simulink model "pv_model_2sx1p_final"  (R2017b)
settings: Solver=ode23tb  StartTime=0.0  StopTime=1.5  MaxStep=1e-4  RelTol=1e-4  AbsTol=1e-5  EnableMultiTasking=on
InitFcn:
  | Nss = str2num(get_param([gcs,'/Nss_'],'Value'));
  | Npp = str2num(get_param([gcs,'/Npp_'],'Value'));
  | G = str2num(get_param([gcs,'/G_'],'Value'));
  | T = str2num(get_param([gcs,'/T_'],'Value'));
  | Rs = Rsn;
  | Rp = (Gn/G)*Rpn;
values from neighbouring files (symbols this model uses):
  a = an    (= 1.3)    [PVCurvePlot_2sx1p.m]
  Gn = 1000    [PVCurvePlot_2sx1p.m]
undefined symbols (not defined in the file or in its folder): a_n, ILn, Iscn, k, Ki, Kv, Ns, q, Rpn, Rsn, T_n, Tn, Vocn
libraries: powerlib x31, simulink x2
settings Model: Creator=marcelo  LastModifiedBy=Ceyhun
settings SolverCC: SolverResetMethod=Robust
settings DataIOCC: LimitDataPoints=on  SaveFormat=Array  SignalLoggingSaveFormat=ModelDataLogs
settings OptimizationCC: ExpressionDepthLimit=2147483647  InitFltsAndDblsToZero=on  LifeSpan=inf
settings DebuggingCC: SaveWithParameterizedLinksMsg=none  UnderspecifiedInitializationDetection=Classic  MergeDetectMultiDrivingBlocksExec=none  SignalResolutionControl=TryResolveAllWithWarning  SolverPrmCheckMsg=warning  FcnCallInpInsideContextMsg=warning  StateNameClashWarn=warning  SFUnexpectedBacktrackingDiag=warning  SFNoUnconditionalDefaultTransitionDiag=warning  SFExecutionAtInitializationDiag=none
settings HardwareCC: ProdBitPerPointer=32  ProdBitPerSizeT=32  ProdBitPerPtrDiffT=32  ProdLargestAtomicFloat=None  ProdIntDivRoundTo=Undefined  ProdEndianess=Unspecified  ProdWordSize=32  ProdHWDeviceType=32-bit Generic
settings ModelReferenceCC: PropagateSignalLabelsOutOfModel=off
settings CodeAppCC: StateflowObjectComments=on
settings GRTTargetCC: TargetFcnLib=ansi_tfl_tmw.mat  TargetLangStandard=C89/C90 (ANSI)  GeneratePreprocessorConditionals=Disable all  CombineOutputUpdateFcns=off  GRTInterface=on
settings ConfigComp: CovMetricSettings=dw  CovHtmlReporting=on  CovSaveCumulativeToWorkspaceVar=on  CovSaveSingleToWorkspaceVar=on  CovExternalEMLEnable=off
settings SimscapeCC: SimscapeNormalizeSystem=off

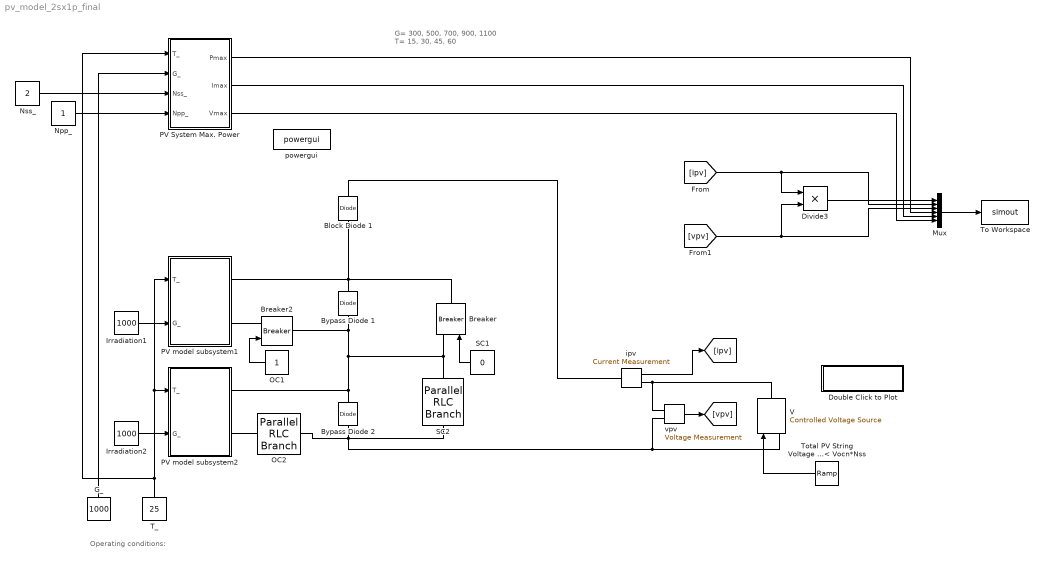
== system pv_model_2sx1p_final ==
  note: G= 300, 500, 700, 900, 1100
      | T= 15, 30, 45, 60
  note: Operating conditions:
  Block Diode 1 : powerlib/Power Electronics/Diode  Ron=0.001  Lon=0  Vf=0.8  IC=0  UseSnubber=off  Rs=500  Cs=250e-9  Measurements=off
  Breaker : powerlib/Elements/Breaker  InitialState=0  SwitchingTimes="[1/60  5/60]"  External=on  BreakerResistance=0.01  SnubberResistance=1e9  SnubberCapacitance=inf  Measurements=None  MoreParameters=on  NoBreakLoop=off
      settings: SourceProductName=Simscape Power Systems
  Breaker2 : powerlib/Elements/Breaker  InitialState=0  SwitchingTimes="[1/60  5/60]"  External=on  BreakerResistance=0.01  SnubberResistance=1e9  SnubberCapacitance=inf  Measurements=None  MoreParameters=on  NoBreakLoop=off
      settings: SourceProductName=Simscape Power Systems
  Bypass Diode 1 : powerlib/Power Electronics/Diode  Ron=0.001  Lon=0  Vf=0.8  IC=0  UseSnubber=off  Rs=500  Cs=250e-9  Measurements=off
  Bypass Diode 2 : powerlib/Power Electronics/Diode  Ron=0.001  Lon=0  Vf=0.8  IC=0  UseSnubber=off  Rs=500  Cs=250e-9  Measurements=off
  Divide3 : Product  Inputs=**
  Double Click to Plot : Subsystem
      settings: OpenFcn=PVCurvePlot_2sx1p
      mask Display: disp('Plot PV Curve');
  G_ : Constant  Value=1000
  Irradiation1 : Constant  Value=1000
  Irradiation2 : Constant  Value=1000
  Mux : Mux  Inputs=6
  Npp_ : Constant
  Nss_ : Constant  Value=2
  OC1 : Constant
  OC2 : powerlib/Elements/Parallel RLC Branch  LConnTagsString=a  RConnTagsString=__new0  BranchType=R  Resistance=0.01  Inductance=1e-3  SetiL0=off  InitialCurrent=0  Capacitance=1e-6  Setx0=off  InitialVoltage=0  Measurements=None
  PV System Max. Power : Subsystem
  PV model subsystem1 : Subsystem
  PV model subsystem2 : Subsystem
  SC1 : Constant  Value=0
  SC2 : powerlib/Elements/Parallel RLC Branch  LConnTagsString=a  RConnTagsString=__new0  BranchType=R  Resistance=1e9  Inductance=1e-3  SetiL0=off  InitialCurrent=0  Capacitance=1e-6  Setx0=off  InitialVoltage=0  Measurements=None
  T_ : Constant  Value=25
  To Workspace : ToWorkspace  VariableName=simout  SampleTime=-1
  Total PV String Voltage 0 < V < Vocn*Nss : simulink/Sources/Ramp  slope=Vocn*2  start=0  X0=0
  V : powerlib/Electrical Sources/Controlled Voltage Source  Initialize=on  Source_Type=DC  Amplitude=0  Phase=0  Frequency=0  Measurements=None
  ipv : powerlib/Measurements/Current Measurement  PhasorSimulation=off  OutputType=Complex  PSBequivalent=0
  powergui : powerlib/powergui  SimulationMode=Continuous  SampleTime=1e-4  frequency=60  Iterations=50  frequencyindice=0  Pbase=100e6  ErrMax=1e-4  UnitsV=kV  UnitsW=MW  buscounter=0  FunctionMessages=off  echomessages=off  EnableUseOfTLC=off  CurrentSourceSwitches=off  DisableSnubberDevices=off  DisableRonSwitches=off  DisableVfSwitches=off  DisplayEquations=off  SolverType=Tustin/Backward Euler (TBE)  Interpol=off  ExternalGateDelay=off  methode=off  Ts=100  x0status=blocks  SPID=on  SwTol=0  HookPort=off  RestoreLinks=warning  ResistiveCurrentMeasurement=off  Frange=[0:2:500]  Ylog=off  Xlog=on  ShowGrid=off  save=off  variable=ZData  structure=0  ZoomFFT=on  StartTime=0.0  cycles=1  DisplayStyle=1  fundamental=60  FreqAxis=off  MaxFrequency=1000  frequencyindicesteady=1  RmsSteady=1  display=off
  vpv : powerlib/Measurements/Voltage Measurement  PhasorSimulation=off  OutputType=Complex  PSBequivalent=0
  wires:
  Total PV String Voltage 0 < V < Vocn*Nss/1 -> V/1
  ipv/1 -> [ipv]
  vpv/1 -> [vpv]
  T_/1 -> PV model subsystem2/1(T_), PV model subsystem1/1(T_), PV System Max. Power/1(T_)
  Irradiation1/1 -> PV model subsystem1/2(G_)
  Irradiation2/1 -> PV model subsystem2/2(G_)
  [ipv] -> Mux/2, Divide3/1
  [vpv] -> Divide3/2, Mux/3
  Divide3/1 -> Mux/1
  Mux/1 -> To Workspace/1
  Nss_/1 -> PV System Max. Power/3(Nss_)
  Npp_/1 -> PV System Max. Power/4(Npp_)
  G_/1 -> PV System Max. Power/2(G_)
  PV System Max. Power/1(Pmax) -> Mux/4
  PV System Max. Power/2(Imax) -> Mux/5
  PV System Max. Power/3(Vmax) -> Mux/6
  SC1/1 -> Breaker/1
  OC1/1 -> Breaker2/1
  connections:
  ipv/RConn1 -- V/RConn1 -- vpv/LConn1
  Bypass Diode 1/RConn1 -- Breaker/RConn1 -- PV model subsystem1/RConn1 -- Block Diode 1/LConn1
  V/LConn1 -- SC2/LConn1 -- OC2/RConn1 -- Bypass Diode 2/LConn1 -- vpv/LConn2
  Bypass Diode 2/RConn1 -- PV model subsystem2/RConn1 -- Breaker2/RConn1 -- Bypass Diode 1/LConn1 -- Breaker/LConn1 -- SC2/RConn1
  Breaker2/LConn1 -- PV model subsystem1/RConn2
  PV model subsystem2/RConn2 -- OC2/LConn1
  Block Diode 1/RConn1 -- ipv/LConn1

== system pv_model_2sx1p_final/Double Click to Plot ==

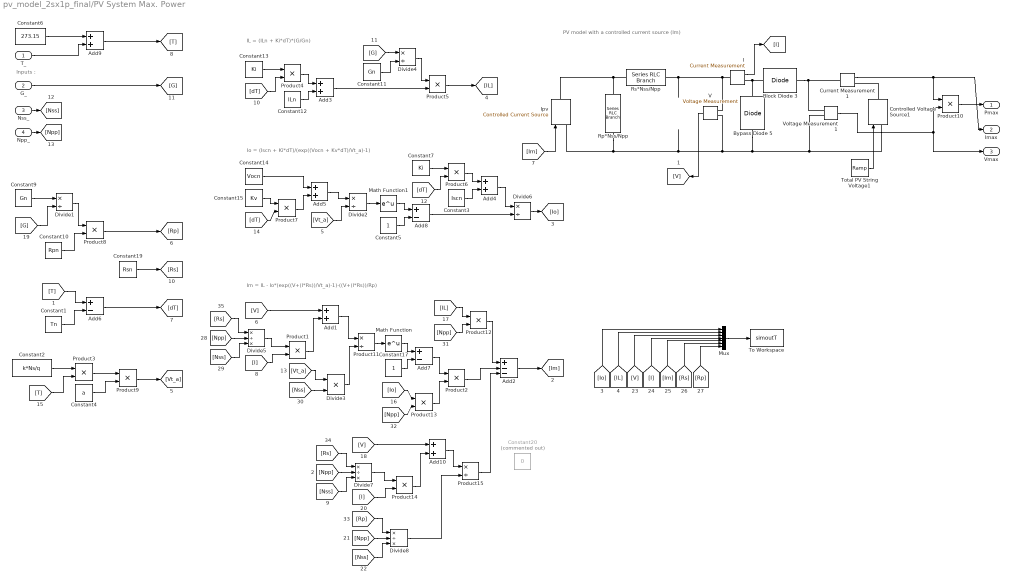
== system pv_model_2sx1p_final/PV System Max. Power ==
  note: Im = IL - Io*(exp((V+(I*Rs))/Vt_a)-1)-((V+(I*Rs))/Rp)
  note: Inputs :
  note: Io = (Iscn + Ki*dT)/(exp((Vocn + Kv*dT)/Vt_a)-1)
  note: PV model with a controlled current source (Im)
  note: IL = (ILn + Ki*dT)*(G/Gn)
  T_ : Inport
  G_ : Inport  Port=2
  Nss_ : Inport  Port=3
  Npp_ : Inport  Port=4
  Add{1,3..5,9..10} (6 alike) : Sum
  Add2 : Sum  Inputs=+--
  Add6 : Sum  Inputs=+-
  Add7 : Sum  Inputs=+-
  Add8 : Sum  Inputs=+-
  Block Diode 3 : powerlib/Power Electronics/Diode  Ron=0.001  Lon=0  Vf=0.8  IC=0  UseSnubber=off  Rs=500  Cs=250e-9  Measurements=off
  Bypass Diode 5 : powerlib/Power Electronics/Diode  Ron=0.001  Lon=0  Vf=0.8  IC=0  UseSnubber=off  Rs=500  Cs=250e-9  Measurements=off
  Constant1 : Constant  Value=Tn
  Constant10 : Constant  Value=Rpn
  Constant11 : Constant  Value=Gn
  Constant12 : Constant  Value=ILn
  Constant13 : Constant  Value=Ki
  Constant14 : Constant  Value=Vocn
  Constant15 : Constant  Value=Kv
  Constant17 : Constant
  Constant19 : Constant  Value=Rsn
  Constant2 : Constant  Value=k*Ns/q
  Constant20 : Constant  Commented=on  Value=0
  Constant3 : Constant  Value=Iscn
  Constant4 : Constant  Value=a
  Constant5 : Constant
  Constant6 : Constant  Value=273.15
  Constant7 : Constant  Value=Ki
  Constant9 : Constant  Value=Gn
  Controlled Voltage Source1 : powerlib/Electrical Sources/Controlled Voltage Source  Initialize=on  Source_Type=DC  Amplitude=0  Phase=0  Frequency=0  Measurements=None
  Current Measurement1 : powerlib/Measurements/Current Measurement  PhasorSimulation=off  OutputType=Complex  PSBequivalent=0
  Divide{1..2,4,6} (4 alike) : Product  Inputs=*/
  Divide3 : Product
  Divide5 : Product  Inputs=*/*
  Divide7 : Product  Inputs=*/*
  Divide8 : Product  Inputs=*/*
  I : powerlib/Measurements/Current Measurement  PhasorSimulation=off  OutputType=Complex  PSBequivalent=0
  Ipv : powerlib/Electrical Sources/Controlled Current Source  Initialize=on  Source_Type=DC  Amplitude=0  Phase=0  Frequency=0  Measurements=None
  Math Function : Math  SaturateOnIntegerOverflow=on
  Math Function1 : Math  SaturateOnIntegerOverflow=on
  Mux : Mux  Inputs=7
  Product{1..9,12..14} (12 alike) : Product  RndMeth=Zero
  Product10 : Product
  Product11 : Product  Inputs=*/  RndMeth=Zero
  Product15 : Product  Inputs=*/  RndMeth=Zero
  Rp*Nss/Npp : powerlib/Elements/Series RLC Branch  LConnTagsString=__new0  RConnTagsString=__new0  BranchType=R  Resistance=Rp*Nss/Npp  Inductance=1e-3  SetiL0=off  InitialCurrent=0  Capacitance=1e-6  Setx0=off  InitialVoltage=0  Measurements=None
  Rs*Nss/Npp : powerlib/Elements/Series RLC Branch  LConnTagsString=__new0  RConnTagsString=__new0  BranchType=R  Resistance=Rs*Nss/Npp  Inductance=1e-3  SetiL0=off  InitialCurrent=0  Capacitance=1e-6  Setx0=off  InitialVoltage=0  Measurements=None
  To Workspace : ToWorkspace  VariableName=simoutT  SampleTime=-1
  Total PV String Voltage1 : simulink/Sources/Ramp  slope=Vocn*Nss  start=0  X0=0
  "V " : powerlib/Measurements/Voltage Measurement  PhasorSimulation=off  OutputType=Complex  PSBequivalent=0
  Voltage Measurement1 : powerlib/Measurements/Voltage Measurement  PhasorSimulation=off  OutputType=Complex  PSBequivalent=0
  Pmax : Outport
  Imax : Outport  Port=2
  Vmax : Outport  Port=3
  wires:
  I/1 -> [I]
  "V "/1 -> [V]
  [Im] -> Ipv/1
  G_/1 -> [G]
  [I] -> Product1/2
  [V] -> Add1/1
  Add2/1 -> [Im]
  [G] -> Divide4/1
  Constant11/1 -> Divide4/2
  Constant13/1 -> Product4/1
  [dT] -> Product6/2
  Constant7/1 -> Product6/1
  [dT] -> Product7/2
  Constant14/1 -> Add5/1
  Divide2/1 -> Math Function1/1
  Add5/1 -> Divide2/1
  Constant17/1 -> Add7/2
  Add7/1 -> Product2/1
  Constant5/1 -> Add8/2
  Math Function1/1 -> Add8/1
  Divide6/1 -> [Io]
  Product5/1 -> [IL]
  Product1/1 -> Add1/2
  Math Function/1 -> Add7/1
  Product4/1 -> Add3/1
  Add3/1 -> Product5/2
  Divide4/1 -> Product5/1
  Product7/1 -> Add5/2
  Constant15/1 -> Product7/1
  Add8/1 -> Divide6/2
  Constant3/1 -> Add4/2
  Product6/1 -> Add4/1
  Constant12/1 -> Add3/2
  Product2/1 -> Add2/2
  [dT] -> Product4/2
  Add4/1 -> Divide6/1
  Mux/1 -> To Workspace/1
  [Io] -> Mux/1
  [IL] -> Mux/2
  Add6/1 -> [dT]
  [T] -> Add6/1
  Constant1/1 -> Add6/2
  Constant2/1 -> Product3/1
  [Rs] -> Mux/6
  Divide1/1 -> Product8/1
  Product8/1 -> [Rp]
  Constant10/1 -> Product8/2
  Add9/1 -> [T]
  [Im] -> Mux/5
  [I] -> Mux/4
  [V] -> Mux/3
  [Vt_a] -> Divide2/2
  Constant4/1 -> Product9/2
  Product3/1 -> Product9/1
  Product9/1 -> [Vt_a]
  [T] -> Product3/2
  Constant9/1 -> Divide1/1
  [G] -> Divide1/2
  T_/1 -> Add9/2
  Constant6/1 -> Add9/1
  [Rp] -> Mux/7
  Constant19/1 -> [Rs]
  [Rs] -> Divide5/1
  Divide5/1 -> Product1/1
  [Npp] -> Divide5/2
  [Nss] -> Divide5/3
  [Vt_a] -> Divide3/1
  [IL] -> Product12/1
  [Npp] -> Product12/2
  Product12/1 -> Add2/1
  [Io] -> Product13/1
  [Npp] -> Product13/2
  Product13/1 -> Product2/2
  Npp_/1 -> [Npp]
  Nss_/1 -> [Nss]
  Voltage Measurement1/1 -> Vmax/1, Product10/2
  Product10/1 -> Pmax/1
  Current Measurement1/1 -> Imax/1, Product10/1
  Total PV String Voltage1/1 -> Controlled Voltage Source1/1
  Product11/1 -> Math Function/1
  Divide3/1 -> Product11/2
  Add1/1 -> Product11/1
  [Nss] -> Divide3/2
  Divide8/1 -> Product15/2
  [Nss] -> Divide7/3
  [Npp] -> Divide7/2
  Product14/1 -> Add10/2
  [I] -> Product14/2
  [Rs] -> Divide7/1
  [V] -> Add10/1
  [Nss] -> Divide8/3
  Divide7/1 -> Product14/1
  Add10/1 -> Product15/1
  [Rp] -> Divide8/1
  [Npp] -> Divide8/2
  Product15/1 -> Add2/3
  connections:
  I/LConn1 -- Rs*Nss/Npp/RConn1 -- "V "/LConn1
  Ipv/RConn1 -- Rs*Nss/Npp/LConn1 -- Rp*Nss/Npp/LConn1
  Controlled Voltage Source1/LConn1 -- Voltage Measurement1/LConn2 -- Bypass Diode 5/LConn1 -- Rp*Nss/Npp/RConn1 -- Ipv/LConn1 -- "V "/LConn2
  Controlled Voltage Source1/RConn1 -- Current Measurement1/RConn1
  Voltage Measurement1/LConn1 -- Current Measurement1/LConn1 -- Block Diode 3/RConn1
  Block Diode 3/LConn1 -- Bypass Diode 5/RConn1 -- I/RConn1

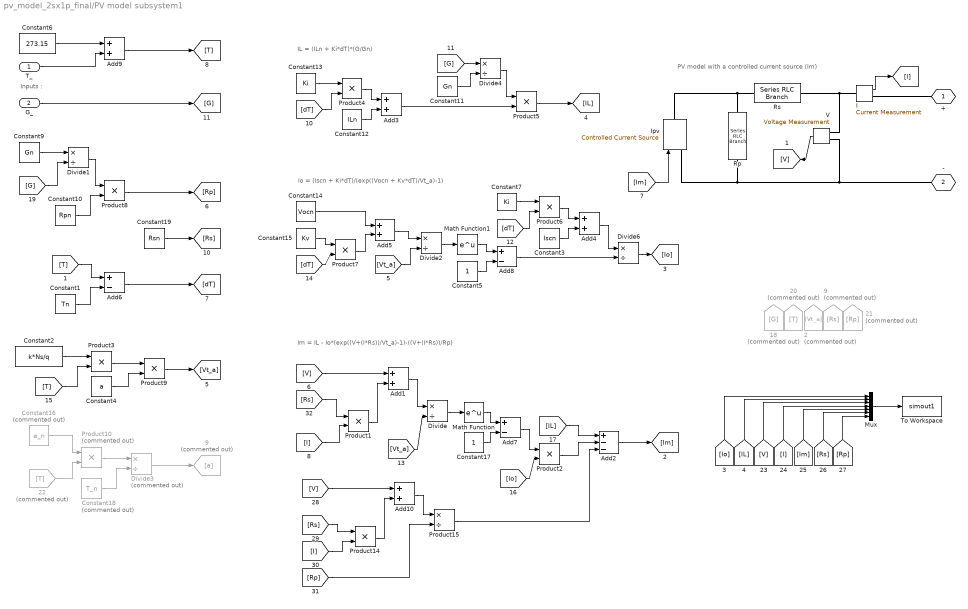
== system pv_model_2sx1p_final/PV model subsystem1 ==
  note: Im = IL - Io*(exp((V+(I*Rs))/Vt_a)-1)-((V+(I*Rs))/Rp)
  note: Inputs :
  note: Io = (Iscn + Ki*dT)/(exp((Vocn + Kv*dT)/Vt_a)-1)
  note: PV model with a controlled current source (Im)
  note: IL = (ILn + Ki*dT)*(G/Gn)
  T_ : Inport
  G_ : Inport  Port=2
  "       9" : Goto  Commented=on  GotoTag=a
  "   18" : From  Commented=on  GotoTag=G
      settings: CloseFcn=tagdialog Close
  "   2" : From  Commented=on  GotoTag=Vt_a
      settings: CloseFcn=tagdialog Close
  "   20" : From  Commented=on  GotoTag=T
      settings: CloseFcn=tagdialog Close
  "   21" : From  Commented=on  GotoTag=Rp
      settings: CloseFcn=tagdialog Close
  "   22" : From  Commented=on  GotoTag=T
      settings: CloseFcn=tagdialog Close
  "   9" : From  Commented=on  GotoTag=Rs
      settings: CloseFcn=tagdialog Close
  Add{1,3..5,9..10} (6 alike) : Sum
  Add2 : Sum  Inputs=+--
  Add6 : Sum  Inputs=+-
  Add7 : Sum  Inputs=+-
  Add8 : Sum  Inputs=+-
  Constant1 : Constant  Value=Tn
  Constant10 : Constant  Value=Rpn
  Constant11 : Constant  Value=Gn
  Constant12 : Constant  Value=ILn
  Constant13 : Constant  Value=Ki
  Constant14 : Constant  Value=Vocn
  Constant15 : Constant  Value=Kv
  Constant16 : Constant  Commented=on  Value=a_n
  Constant17 : Constant
  Constant18 : Constant  Commented=on  Value=T_n
  Constant19 : Constant  Value=Rsn
  Constant2 : Constant  Value=k*Ns/q
  Constant3 : Constant  Value=Iscn
  Constant4 : Constant  Value=a
  Constant5 : Constant
  Constant6 : Constant  Value=273.15
  Constant7 : Constant  Value=Ki
  Constant9 : Constant  Value=Gn
  Divide{,1..2,4,6} (5 alike) : Product  Inputs=*/
  Divide3 : Product  Commented=on  Inputs=*/
  I : powerlib/Measurements/Current Measurement  PhasorSimulation=off  OutputType=Complex  PSBequivalent=0
  Ipv : powerlib/Electrical Sources/Controlled Current Source  Initialize=on  Source_Type=DC  Amplitude=0  Phase=0  Frequency=0  Measurements=None
  Math Function : Math  SaturateOnIntegerOverflow=on
  Math Function1 : Math  SaturateOnIntegerOverflow=on
  Mux : Mux  Inputs=7
  Product{1..9,14} (10 alike) : Product  RndMeth=Zero
  Product10 : Product  Commented=on  RndMeth=Zero
  Product15 : Product  Inputs=*/  RndMeth=Zero
  Rp : powerlib/Elements/Series RLC Branch  LConnTagsString=__new0  RConnTagsString=__new0  BranchType=R  Resistance=Rp  Inductance=1e-3  SetiL0=off  InitialCurrent=0  Capacitance=1e-6  Setx0=off  InitialVoltage=0  Measurements=None
  Rs : powerlib/Elements/Series RLC Branch  LConnTagsString=__new0  RConnTagsString=__new0  BranchType=R  Resistance=Rs  Inductance=1e-3  SetiL0=off  InitialCurrent=0  Capacitance=1e-6  Setx0=off  InitialVoltage=0  Measurements=None
  To Workspace : ToWorkspace  VariableName=simout1  SampleTime=-1
  "V " : powerlib/Measurements/Voltage Measurement  PhasorSimulation=off  OutputType=Complex  PSBequivalent=0
  + : PMIOPort  Port=1  Side=Right
  - : PMIOPort  Port=2  Side=Right
  wires:
  I/1 -> [I]
  "V "/1 -> [V]
  [Im] -> Ipv/1
  G_/1 -> [G]
  [I] -> Product1/2
  [V] -> Add1/1
  Divide/1 -> Math Function/1
  Add2/1 -> [Im]
  Add1/1 -> Divide/1
  [G] -> Divide4/1
  Constant11/1 -> Divide4/2
  Constant13/1 -> Product4/1
  [dT] -> Product6/2
  Constant7/1 -> Product6/1
  [dT] -> Product7/2
  Constant14/1 -> Add5/1
  Divide2/1 -> Math Function1/1
  Add5/1 -> Divide2/1
  Constant17/1 -> Add7/2
  Add7/1 -> Product2/1
  Constant5/1 -> Add8/2
  Math Function1/1 -> Add8/1
  Divide6/1 -> [Io]
  Product5/1 -> [IL]
  Product1/1 -> Add1/2
  Math Function/1 -> Add7/1
  Product4/1 -> Add3/1
  Add3/1 -> Product5/2
  Divide4/1 -> Product5/1
  Product7/1 -> Add5/2
  Constant15/1 -> Product7/1
  Add8/1 -> Divide6/2
  Constant3/1 -> Add4/2
  Product6/1 -> Add4/1
  Constant12/1 -> Add3/2
  Product2/1 -> Add2/2
  [Io] -> Product2/2
  [IL] -> Add2/1
  [Rs] -> Product1/1
  [dT] -> Product4/2
  Add4/1 -> Divide6/1
  Mux/1 -> To Workspace/1
  [Io] -> Mux/1
  [IL] -> Mux/2
  Add6/1 -> [dT]
  [T] -> Add6/1
  Constant1/1 -> Add6/2
  Constant2/1 -> Product3/1
  [Rs] -> Mux/6
  Divide1/1 -> Product8/1
  Product8/1 -> [Rp]
  Constant10/1 -> Product8/2
  Add9/1 -> [T]
  [Im] -> Mux/5
  [I] -> Mux/4
  [V] -> Mux/3
  [Vt_a] -> Divide2/2
  [Vt_a] -> Divide/2
  Constant4/1 -> Product9/2
  Product3/1 -> Product9/1
  Product9/1 -> [Vt_a]
  [T] -> Product3/2
  Constant9/1 -> Divide1/1
  [G] -> Divide1/2
  T_/1 -> Add9/2
  Constant6/1 -> Add9/1
  Constant16/1 -> Product10/1
  "   22"/1 -> Product10/2
  Product10/1 -> Divide3/1
  Constant18/1 -> Divide3/2
  Divide3/1 -> "       9"/1
  [Rp] -> Mux/7
  Constant19/1 -> [Rs]
  [Rp] -> Product15/2
  Product14/1 -> Add10/2
  [I] -> Product14/2
  [V] -> Add10/1
  [Rs] -> Product14/1
  Product15/1 -> Add2/3
  Add10/1 -> Product15/1
  connections:
  I/LConn1 -- "V "/LConn1 -- Rs/RConn1
  -/RConn1 -- Rp/RConn1 -- Ipv/LConn1 -- "V "/LConn2
  +/RConn1 -- I/RConn1
  Ipv/RConn1 -- Rs/LConn1 -- Rp/LConn1

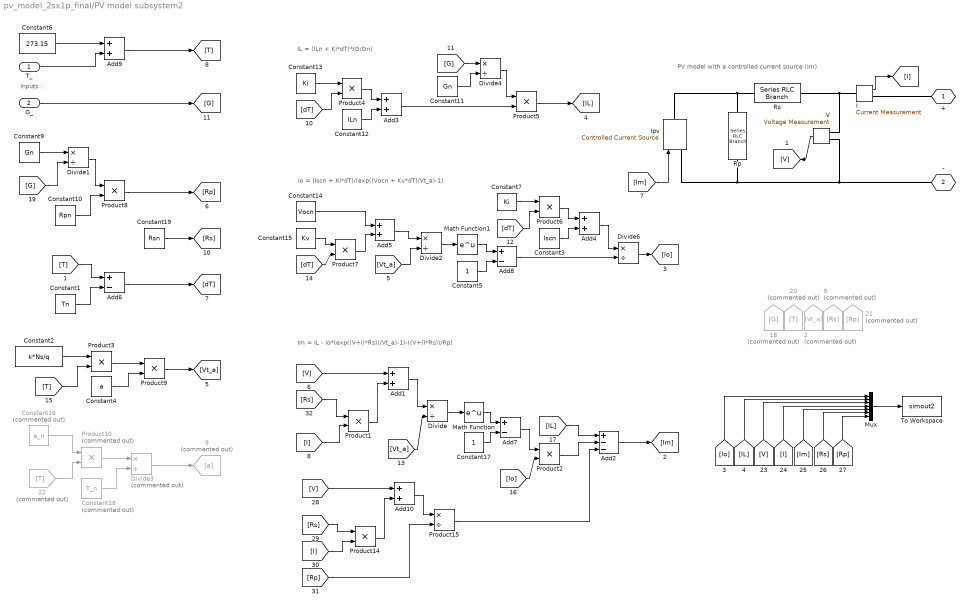
== system pv_model_2sx1p_final/PV model subsystem2 ==
  note: Im = IL - Io*(exp((V+(I*Rs))/Vt_a)-1)-((V+(I*Rs))/Rp)
  note: Inputs :
  note: Io = (Iscn + Ki*dT)/(exp((Vocn + Kv*dT)/Vt_a)-1)
  note: PV model with a controlled current source (Im)
  note: IL = (ILn + Ki*dT)*(G/Gn)
  T_ : Inport
  G_ : Inport  Port=2
  "       9" : Goto  Commented=on  GotoTag=a
  "   18" : From  Commented=on  GotoTag=G
      settings: CloseFcn=tagdialog Close
  "   2" : From  Commented=on  GotoTag=Vt_a
      settings: CloseFcn=tagdialog Close
  "   20" : From  Commented=on  GotoTag=T
      settings: CloseFcn=tagdialog Close
  "   21" : From  Commented=on  GotoTag=Rp
      settings: CloseFcn=tagdialog Close
  "   22" : From  Commented=on  GotoTag=T
      settings: CloseFcn=tagdialog Close
  "   9" : From  Commented=on  GotoTag=Rs
      settings: CloseFcn=tagdialog Close
  Add{1,3..5,9..10} (6 alike) : Sum
  Add2 : Sum  Inputs=+--
  Add6 : Sum  Inputs=+-
  Add7 : Sum  Inputs=+-
  Add8 : Sum  Inputs=+-
  Constant1 : Constant  Value=Tn
  Constant10 : Constant  Value=Rpn
  Constant11 : Constant  Value=Gn
  Constant12 : Constant  Value=ILn
  Constant13 : Constant  Value=Ki
  Constant14 : Constant  Value=Vocn
  Constant15 : Constant  Value=Kv
  Constant16 : Constant  Commented=on  Value=a_n
  Constant17 : Constant
  Constant18 : Constant  Commented=on  Value=T_n
  Constant19 : Constant  Value=Rsn
  Constant2 : Constant  Value=k*Ns/q
  Constant3 : Constant  Value=Iscn
  Constant4 : Constant  Value=a
  Constant5 : Constant
  Constant6 : Constant  Value=273.15
  Constant7 : Constant  Value=Ki
  Constant9 : Constant  Value=Gn
  Divide{,1..2,4,6} (5 alike) : Product  Inputs=*/
  Divide3 : Product  Commented=on  Inputs=*/
  I : powerlib/Measurements/Current Measurement  PhasorSimulation=off  OutputType=Complex  PSBequivalent=0
  Ipv : powerlib/Electrical Sources/Controlled Current Source  Initialize=on  Source_Type=DC  Amplitude=0  Phase=0  Frequency=0  Measurements=None
  Math Function : Math  SaturateOnIntegerOverflow=on
  Math Function1 : Math  SaturateOnIntegerOverflow=on
  Mux : Mux  Inputs=7
  Product{1..9,14} (10 alike) : Product  RndMeth=Zero
  Product10 : Product  Commented=on  RndMeth=Zero
  Product15 : Product  Inputs=*/  RndMeth=Zero
  Rp : powerlib/Elements/Series RLC Branch  LConnTagsString=__new0  RConnTagsString=__new0  BranchType=R  Resistance=Rp  Inductance=1e-3  SetiL0=off  InitialCurrent=0  Capacitance=1e-6  Setx0=off  InitialVoltage=0  Measurements=None
  Rs : powerlib/Elements/Series RLC Branch  LConnTagsString=__new0  RConnTagsString=__new0  BranchType=R  Resistance=Rs  Inductance=1e-3  SetiL0=off  InitialCurrent=0  Capacitance=1e-6  Setx0=off  InitialVoltage=0  Measurements=None
  To Workspace : ToWorkspace  VariableName=simout2  SampleTime=-1
  "V " : powerlib/Measurements/Voltage Measurement  PhasorSimulation=off  OutputType=Complex  PSBequivalent=0
  + : PMIOPort  Port=1  Side=Right
  - : PMIOPort  Port=2  Side=Right
  wires:
  I/1 -> [I]
  "V "/1 -> [V]
  [Im] -> Ipv/1
  G_/1 -> [G]
  [I] -> Product1/2
  [V] -> Add1/1
  Divide/1 -> Math Function/1
  Add2/1 -> [Im]
  Add1/1 -> Divide/1
  [G] -> Divide4/1
  Constant11/1 -> Divide4/2
  Constant13/1 -> Product4/1
  [dT] -> Product6/2
  Constant7/1 -> Product6/1
  [dT] -> Product7/2
  Constant14/1 -> Add5/1
  Divide2/1 -> Math Function1/1
  Add5/1 -> Divide2/1
  Constant17/1 -> Add7/2
  Add7/1 -> Product2/1
  Constant5/1 -> Add8/2
  Math Function1/1 -> Add8/1
  Divide6/1 -> [Io]
  Product5/1 -> [IL]
  Product1/1 -> Add1/2
  Math Function/1 -> Add7/1
  Product4/1 -> Add3/1
  Add3/1 -> Product5/2
  Divide4/1 -> Product5/1
  Product7/1 -> Add5/2
  Constant15/1 -> Product7/1
  Add8/1 -> Divide6/2
  Constant3/1 -> Add4/2
  Product6/1 -> Add4/1
  Constant12/1 -> Add3/2
  Product2/1 -> Add2/2
  [Io] -> Product2/2
  [IL] -> Add2/1
  [Rs] -> Product1/1
  [dT] -> Product4/2
  Add4/1 -> Divide6/1
  Mux/1 -> To Workspace/1
  [Io] -> Mux/1
  [IL] -> Mux/2
  Add6/1 -> [dT]
  [T] -> Add6/1
  Constant1/1 -> Add6/2
  Constant2/1 -> Product3/1
  [Rs] -> Mux/6
  Divide1/1 -> Product8/1
  Product8/1 -> [Rp]
  Constant10/1 -> Product8/2
  Add9/1 -> [T]
  [Im] -> Mux/5
  [I] -> Mux/4
  [V] -> Mux/3
  [Vt_a] -> Divide2/2
  [Vt_a] -> Divide/2
  Constant4/1 -> Product9/2
  Product3/1 -> Product9/1
  Product9/1 -> [Vt_a]
  [T] -> Product3/2
  Constant9/1 -> Divide1/1
  [G] -> Divide1/2
  T_/1 -> Add9/2
  Constant6/1 -> Add9/1
  Constant16/1 -> Product10/1
  "   22"/1 -> Product10/2
  Product10/1 -> Divide3/1
  Constant18/1 -> Divide3/2
  Divide3/1 -> "       9"/1
  [Rp] -> Mux/7
  Constant19/1 -> [Rs]
  [Rp] -> Product15/2
  Product14/1 -> Add10/2
  [I] -> Product14/2
  [V] -> Add10/1
  [Rs] -> Product14/1
  Product15/1 -> Add2/3
  Add10/1 -> Product15/1
  connections:
  I/LConn1 -- "V "/LConn1 -- Rs/RConn1
  -/RConn1 -- Rp/RConn1 -- Ipv/LConn1 -- "V "/LConn2
  +/RConn1 -- I/RConn1
  Ipv/RConn1 -- Rs/LConn1 -- Rp/LConn1
